simulink model "slvv_reqlink"  (R2015b)
settings: Solver=FixedStepDiscrete  SolverMode=SingleTasking  StartTime=0.0  StopTime=10  RelTol=1e-3
libraries: simulink x1
settings Model: Creator=at-mt  LastModifiedBy=amatsumo
settings DataIOCC: SaveFormat=Array  SignalLoggingSaveFormat=ModelDataLogs  SaveOutput=off  SignalLogging=off  SaveTime=off
settings OptimizationCC: BlockReduction=off  ConditionallyExecuteInputs=off  DefaultParameterBehavior=Inlined  ExpressionDepthLimit=2147483647
settings DebuggingCC: AlgebraicLoopMsg=error  UnderspecifiedInitializationDetection=Classic  MergeDetectMultiDrivingBlocksExec=none  SolverPrmCheckMsg=warning  SingleTaskRateTransMsg=error  FcnCallInpInsideContextMsg=UseLocalSettings  StateNameClashWarn=warning
settings HardwareCC: ProdBitPerPointer=32  ProdLargestAtomicFloat=None  ProdIntDivRoundTo=Undefined  ProdEndianess=Unspecified  ProdWordSize=32  ProdHWDeviceType=ASIC/FPGA->ASIC/FPGA  ProdEqTarget=off
settings SFSimCC: SFSimEcho=off  SimParseCustomCode=off
settings GRTTargetCC: GeneratePreprocessorConditionals=Disable all  CombineOutputUpdateFcns=off  GRTInterface=on
settings ConfigComp: RecordCoverage=on  CovPath=small_controller  CovMetricSettings=dcmtrzw  CovHTMLOptions=-sRT=1 -sVT=0 -aTS=1 -bRG=1 -bTC=1 -hTR=0 -nFC=0 -nFD=1 -scm=1 -bcm=1 -xEv=0 -xEM=0  CovSFcnEnable=off

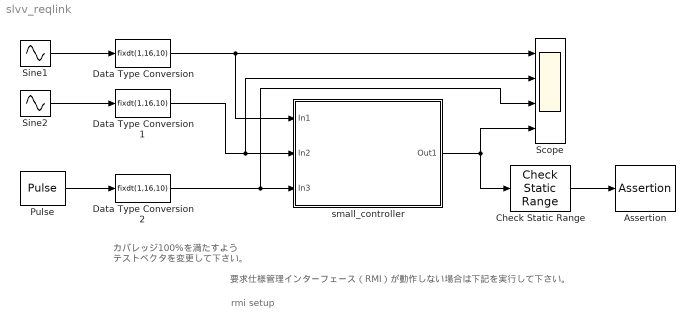
== system slvv_reqlink ==
  note: rmi setup
  note: 要求仕様管理インターフェース（RMI）が動作しない場合は下記を実行して下さい。
  note: カバレッジ100%を満たすよう
      | テストベクタを変更して下さい。
  Assertion : Assertion
  Check Static Range : simulink/Model Verification/Check  Static Range  Description=-0.5 <= u <= 0.5  max=0.5  max_included=on  min=-0.5  min_included=on  enabled=on  stopWhenAssertionFail=on  export=on  icon=graphic
  Data Type Conversion : DataTypeConversion  OutMax=8.5  OutDataTypeStr=fixdt(1,16,10)
  Data Type Conversion1 : DataTypeConversion  OutMax=8.5  OutDataTypeStr=fixdt(1,16,10)
  Data Type Conversion2 : DataTypeConversion  OutDataTypeStr=fixdt(1,16,10)
  Pulse : DiscretePulseGenerator  Period=10  PulseWidth=5  SampleTime=0.1
  Scope : Scope  NumInputPorts=4
  Sine1 : Sin  Amplitude=4  Bias=0 %6  Frequency=0.5*2*pi  SampleTime=0.1
  Sine2 : Sin  Amplitude=4  Bias=6  Frequency=0.2*2*pi  Phase=pi/2  SampleTime=0.1
  small_controller : Subsystem  RequirementInfo={} %GIDa_0ad06f01_c5fa_4905_9abd_571366dd2316
  wires:
  Pulse/1 -> Data Type Conversion2/1
  Sine1/1 -> Data Type Conversion/1
  Sine2/1 -> Data Type Conversion1/1
  Data Type Conversion/1 -> small_controller/1(In1), Scope/1
  Data Type Conversion1/1 -> small_controller/2(In2), Scope/2
  Data Type Conversion2/1 -> small_controller/3(In3), Scope/3
  small_controller/1(Out1) -> Scope/4, Check Static Range/1
  Check Static Range/1 -> Assertion/1

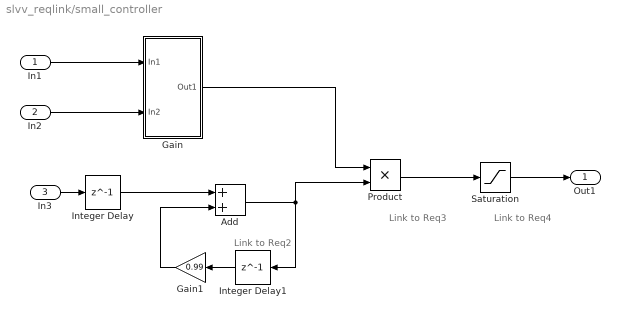
== system slvv_reqlink/small_controller ==
  note: Link to Req4
  note: Link to Req3
  note: Link to Req2
  In1 : Inport
  In2 : Inport  Port=2
  In3 : Inport  Port=3
  Add : Sum  RequirementInfo={'other' 'requirement_sample1.xls' '@Simulink_requirement_item_2' 'true' 'Req2' '' } %GIDa_2e34b87f_d780_43c2_b42f_38c8a4001266  OutDataTypeStr=Inherit: Same as first input
  Gain : Subsystem
  Gain1 : Gain  Gain=0.99
  Integer Delay : Delay  DelayLength=1  InputProcessing=Inherited
  Integer Delay1 : Delay  RequirementInfo={} %GIDa_536ab486_8ad1_4363_ac83_15cad1d4f43e  DelayLength=1  InputProcessing=Inherited
  Product : Product  RequirementInfo={'other' 'requirement_sample1.xls' '@Simulink_requirement_item_3' 'true' 'Req3' '' } %GIDa_40bd7063_4109_4539_bda3_85cd9a729e74  RndMeth=Zero
  Saturation : Saturate  RequirementInfo={'other' 'requirement_sample1.xls' '@Simulink_requirement_item_4' 'true' 'Req4' '' } %GIDa_330285bc_4120_41bf_962d_d8c5df303a45
  Out1 : Outport
  wires:
  Product/1 -> Saturation/1
  Gain/1(Out1) -> Product/1
  In1/1 -> Gain/1(In1)
  In2/1 -> Gain/2(In2)
  Saturation/1 -> Out1/1
  In3/1 -> Integer Delay/1
  Integer Delay/1 -> Add/1
  Integer Delay1/1 -> Gain1/1
  Add/1 -> Integer Delay1/1, Product/2
  Gain1/1 -> Add/2

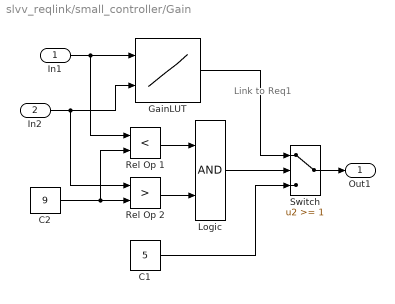
== system slvv_reqlink/small_controller/Gain ==
  note: Link to Req1
  In1 : Inport
  In2 : Inport  Port=2
  C1 : Constant  Value=5  OutDataTypeStr=fixdt(1,16,10)
  C2 : Constant  Value=9  OutDataTypeStr=fixdt(1,16,10)
  GainLUT : Lookup_n-D  RequirementInfo={'other' 'requirement_sample1.xls' '@Simulink_requirement_item_1' 'true' 'Req1' '' } %GIDa_34cc6e4e_ead7_4e76_b3ee_8a30591f460c  BreakpointsForDimension1=[1:0.25:10]  BreakpointsForDimension2=[1:0.25:10]  IndexSearchMethod=Evenly spaced points  Table=sqrt([1:0.25:10]'*[1:0.25:10])  InterpMethod=Flat  InputSameDT=on
  Logic : Logic  AllPortsSameDT=off  OutDataTypeStr=boolean
  Rel Op 1 : RelationalOperator  Operator=<  OutDataTypeStr=boolean
  Rel Op 2 : RelationalOperator  Operator=>  OutDataTypeStr=boolean
  Switch : Switch  Threshold=1
  Out1 : Outport
  wires:
  Switch/1 -> Out1/1
  Rel Op 2/1 -> Logic/2
  Rel Op 1/1 -> Logic/1
  C2/1 -> Rel Op 1/2, Rel Op 2/2
  Logic/1 -> Switch/2
  In2/1 -> Rel Op 2/1, GainLUT/2
  In1/1 -> Rel Op 1/1, GainLUT/1
  GainLUT/1 -> Switch/1
  C1/1 -> Switch/3
